simulink model "counter_direction"  (R2017a)
settings: Solver=FixedStepDiscrete  StartTime=0.0  StopTime=500000  FixedStep=1  RelTol=1e-3
libraries: hdlsllib x14, simulink x3
settings Model: Creator=Patrick  LastModifiedBy=wachala.j
settings OptimizationCC: BlockReduction=off  ConditionallyExecuteInputs=off  DefaultParameterBehavior=Inlined
settings DebuggingCC: AlgebraicLoopMsg=error
settings HardwareCC: ProdBitPerPointer=32  ProdBitPerSizeT=32  ProdBitPerPtrDiffT=32  ProdLargestAtomicFloat=None  ProdIntDivRoundTo=Undefined  ProdEndianess=Unspecified  ProdWordSize=32  ProdHWDeviceType=ASIC/FPGA->ASIC/FPGA  ProdEqTarget=off
settings SFSimCC: SimUseLocalCustomCode=on
settings RTWCC: RTWUseLocalCustomCode=on

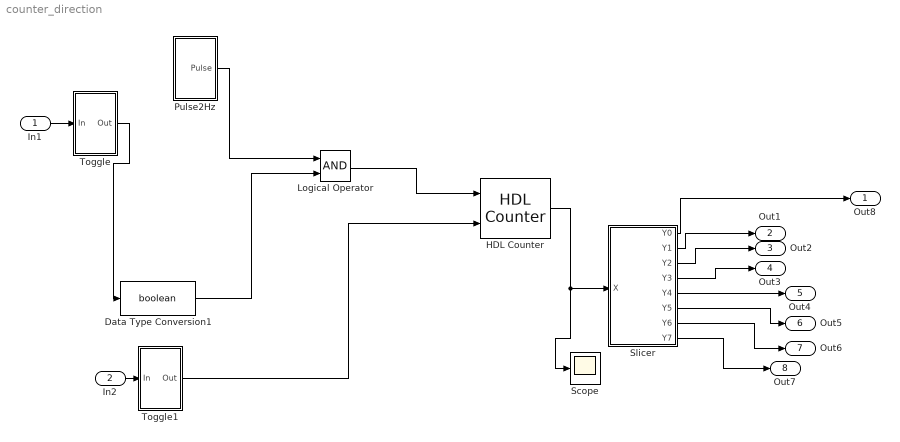
== system counter_direction ==
  In1 : Inport
  In2 : Inport  Port=2
  Data Type Conversion1 : DataTypeConversion  OutDataTypeStr=boolean
  HDL Counter : hdlsllib/HDL Operations/HDL Counter  CountType=Free running  CountInit=0  CountStep=1  CountMax=255  CountFromType=Initial value  CountFrom=0  CountResetPort=off  CountLoadPort=off  CountEnbPort=on  CountDirPort=on  CountDataType=Unsigned  CountWordLen=8  CountFracLen=0  CountSampTime=1
      settings: SourceProductName=HDL Coder  SourceProductBaseCode=HD
  Logical Operator : Logic  AllPortsSameDT=off  OutDataTypeStr=boolean
  Pulse2Hz : Subsystem
  Scope : Scope
  Slicer : Subsystem
  Toggle : Subsystem
  Toggle1 : Subsystem
  Out8 : Outport
  Out1 : Outport  Port=2
  Out2 : Outport  Port=3
  Out3 : Outport  Port=4
  Out4 : Outport  Port=5
  Out5 : Outport  Port=6
  Out6 : Outport  Port=7
  Out7 : Outport  Port=8
  wires:
  Slicer/1(Y0) -> Out8/1
  Slicer/2(Y1) -> Out1/1
  Slicer/4(Y3) -> Out3/1
  Slicer/6(Y5) -> Out5/1
  Slicer/5(Y4) -> Out4/1
  Slicer/3(Y2) -> Out2/1
  Slicer/8(Y7) -> Out7/1
  Slicer/7(Y6) -> Out6/1
  HDL Counter/1 -> Scope/1, Slicer/1(X)
  Toggle/1(Out) -> Data Type Conversion1/1
  Logical Operator/1 -> HDL Counter/1
  Data Type Conversion1/1 -> Logical Operator/2
  Toggle1/1(Out) -> HDL Counter/2
  Pulse2Hz/1(Pulse) -> Logical Operator/1
  In1/1 -> Toggle/1(In)
  In2/1 -> Toggle1/1(In)

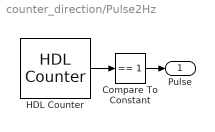
== system counter_direction/Pulse2Hz ==
  Compare To Constant : simulink/Logic and Bit Operations/Compare To Constant  relop===  const=1  OutDataTypeStr=boolean
  HDL Counter : hdlsllib/HDL Operations/HDL Counter  CountType=Count limited  CountInit=0  CountStep=1  CountMax=25000000  CountFromType=Initial value  CountFrom=0  CountResetPort=off  CountLoadPort=off  CountEnbPort=off  CountDirPort=off  CountDataType=Unsigned  CountWordLen=32  CountFracLen=0  CountSampTime=1
      settings: SourceProductName=HDL Coder  SourceProductBaseCode=HD
  Pulse : Outport
  wires:
  HDL Counter/1 -> Compare To Constant/1
  Compare To Constant/1 -> Pulse/1

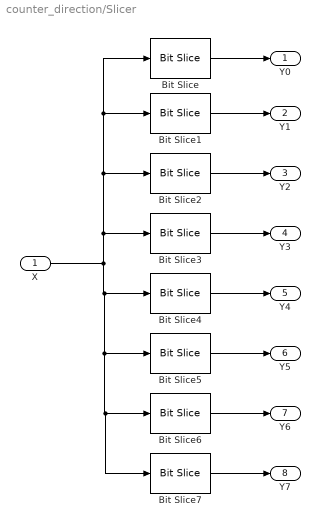
== system counter_direction/Slicer ==
  X : Inport  OutDataTypeStr=uint8  SampleTime=1
  Bit Slice : hdlsllib/HDL Operations/Bit Slice  lidx=7  ridx=7
      settings: SourceProductName=HDL Coder  SourceProductBaseCode=HD
  Bit Slice1 : hdlsllib/HDL Operations/Bit Slice  lidx=6  ridx=6
      settings: SourceProductName=HDL Coder  SourceProductBaseCode=HD
  Bit Slice2 : hdlsllib/HDL Operations/Bit Slice  lidx=5  ridx=5
      settings: SourceProductName=HDL Coder  SourceProductBaseCode=HD
  Bit Slice3 : hdlsllib/HDL Operations/Bit Slice  lidx=4  ridx=4
      settings: SourceProductName=HDL Coder  SourceProductBaseCode=HD
  Bit Slice4 : hdlsllib/HDL Operations/Bit Slice  lidx=3  ridx=3
      settings: SourceProductName=HDL Coder  SourceProductBaseCode=HD
  Bit Slice5 : hdlsllib/HDL Operations/Bit Slice  lidx=2  ridx=2
      settings: SourceProductName=HDL Coder  SourceProductBaseCode=HD
  Bit Slice6 : hdlsllib/HDL Operations/Bit Slice  lidx=1  ridx=1
      settings: SourceProductName=HDL Coder  SourceProductBaseCode=HD
  Bit Slice7 : hdlsllib/HDL Operations/Bit Slice  lidx=0  ridx=0
      settings: SourceProductName=HDL Coder  SourceProductBaseCode=HD
  Y0 : Outport
  Y1 : Outport  Port=2
  Y2 : Outport  Port=3
  Y3 : Outport  Port=4
  Y4 : Outport  Port=5
  Y5 : Outport  Port=6
  Y6 : Outport  Port=7
  Y7 : Outport  Port=8
  wires:
  Bit Slice1/1 -> Y1/1
  Bit Slice7/1 -> Y7/1
  X/1 -> Bit Slice7/1, Bit Slice6/1, Bit Slice5/1, Bit Slice4/1, Bit Slice3/1, Bit Slice2/1, Bit Slice1/1, Bit Slice/1
  Bit Slice/1 -> Y0/1
  Bit Slice4/1 -> Y4/1
  Bit Slice2/1 -> Y2/1
  Bit Slice5/1 -> Y5/1
  Bit Slice3/1 -> Y3/1
  Bit Slice6/1 -> Y6/1

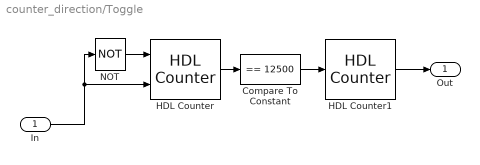
== system counter_direction/Toggle ==
  In : Inport  OutDataTypeStr=boolean
  Compare To Constant : simulink/Logic and Bit Operations/Compare To Constant  relop===  const=12500  OutDataTypeStr=boolean
  HDL Counter : hdlsllib/HDL Operations/HDL Counter  CountType=Count limited  CountInit=0  CountStep=1  CountMax=50000000  CountFromType=Initial value  CountFrom=0  CountResetPort=on  CountLoadPort=off  CountEnbPort=on  CountDirPort=off  CountDataType=Unsigned  CountWordLen=50  CountFracLen=0  CountSampTime=1
      settings: SourceProductName=HDL Coder  SourceProductBaseCode=HD
  HDL Counter1 : hdlsllib/HDL Operations/HDL Counter  CountType=Free running  CountInit=0  CountStep=1  CountMax=25  CountFromType=Initial value  CountFrom=0  CountResetPort=off  CountLoadPort=off  CountEnbPort=on  CountDirPort=off  CountDataType=Unsigned  CountWordLen=1  CountFracLen=0  CountSampTime=1
      settings: SourceProductName=HDL Coder  SourceProductBaseCode=HD
  NOT : Logic  Operator=NOT  IconShape=distinctive  AllPortsSameDT=off  OutDataTypeStr=boolean
  Out : Outport  SampleTime=1
  wires:
  HDL Counter/1 -> Compare To Constant/1
  Compare To Constant/1 -> HDL Counter1/1
  NOT/1 -> HDL Counter/1
  HDL Counter1/1 -> Out/1
  In/1 -> NOT/1, HDL Counter/2

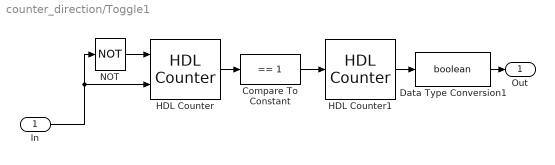
== system counter_direction/Toggle1 ==
  In : Inport  OutDataTypeStr=boolean
  Compare To Constant : simulink/Logic and Bit Operations/Compare To Constant  relop===  const=1  OutDataTypeStr=boolean
  Data Type Conversion1 : DataTypeConversion  OutDataTypeStr=boolean
  HDL Counter : hdlsllib/HDL Operations/HDL Counter  CountType=Count limited  CountInit=0  CountStep=1  CountMax=50000000  CountFromType=Initial value  CountFrom=0  CountResetPort=on  CountLoadPort=off  CountEnbPort=on  CountDirPort=off  CountDataType=Unsigned  CountWordLen=50  CountFracLen=0  CountSampTime=1
      settings: SourceProductName=HDL Coder  SourceProductBaseCode=HD
  HDL Counter1 : hdlsllib/HDL Operations/HDL Counter  CountType=Free running  CountInit=0  CountStep=1  CountMax=25  CountFromType=Initial value  CountFrom=0  CountResetPort=off  CountLoadPort=off  CountEnbPort=on  CountDirPort=off  CountDataType=Unsigned  CountWordLen=1  CountFracLen=0  CountSampTime=1
      settings: SourceProductName=HDL Coder  SourceProductBaseCode=HD
  NOT : Logic  Operator=NOT  IconShape=distinctive  AllPortsSameDT=off  OutDataTypeStr=boolean
  Out : Outport  SampleTime=1
  wires:
  HDL Counter/1 -> Compare To Constant/1
  Compare To Constant/1 -> HDL Counter1/1
  NOT/1 -> HDL Counter/1
  In/1 -> NOT/1, HDL Counter/2
  HDL Counter1/1 -> Data Type Conversion1/1
  Data Type Conversion1/1 -> Out/1
